simulink model "Linear_sys"  (R2024b)
settings: Solver=VariableStepAuto  StartTime=0.0  StopTime=300  RelTol=1e-3
settings Model: Creator=shalh  LastModifiedBy=shalh

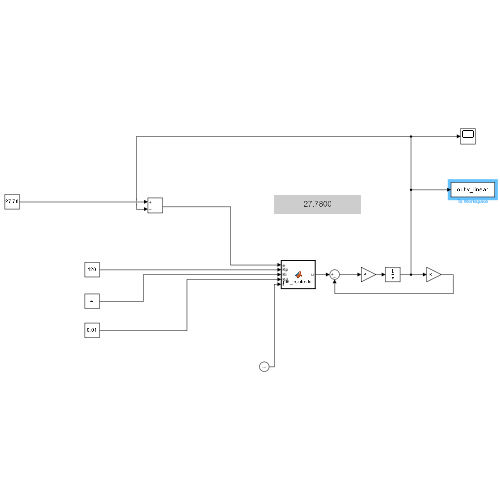
[thumbnail: Simulink's stored preview of the top-level diagram]
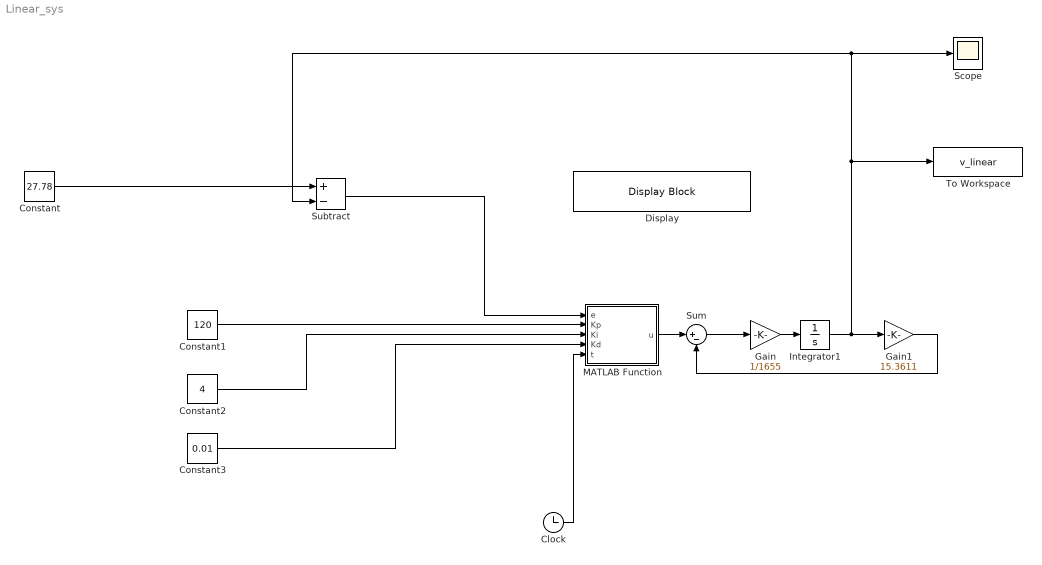
== system Linear_sys ==
  Clock : Clock
      settings: Decimation=40
  Constant : Constant  Value=27.78
  Constant1 : Constant  Value=120
  Constant2 : Constant  Value=4
  Constant3 : Constant  Value=0.01
  Display : DisplayBlock  LabelPosition=Hide  Transparency=1
  Gain : Gain  Gain=1/1655
  Gain1 : Gain  Gain=15.3611
  Integrator1 : Integrator
  MATLAB Function : MATLAB Function  TreatAsAtomicUnit=on
  Scope : Scope
  Subtract : Sum  Inputs=+-
  Sum : Sum  Inputs=|+-
  To Workspace : ToWorkspace  VariableName=v_linear  SampleTime=-1
  wires:
  Gain1/1 -> Sum/2
  Sum/1 -> Gain/1
  Constant3/1 -> MATLAB Function/4(Kd)
  Clock/1 -> MATLAB Function/5(t)
  Gain/1 -> Integrator1/1
  Subtract/1 -> MATLAB Function/1(e)
  Constant2/1 -> MATLAB Function/3(Ki)
  Constant1/1 -> MATLAB Function/2(Kp)
  MATLAB Function/1(u) -> Sum/1
  Constant/1 -> Subtract/1
  Integrator1/1 -> Scope/1, Subtract/2, To Workspace/1, Gain1/1

== matlab function Linear_sys/MATLAB Function ==
  settings: updateMethod=DISCRETE
  data: e input double; Kp input; Ki input; Kd input; u output double; t input
function u = pid_controller(e,Kp,Ki, Kd, t)
  
    persistent e_integral e_prev t_prev
    if isempty(e_integral)
        e_integral = 0;
        e_prev = 0;
        t_prev = 0;
    end
    
    
    if t_prev == 0
        dt = 0.01; 
    else
        dt = t - t_prev;
    end
    
    e_integral = e_integral + e * dt;
    
    if dt > 0
        e_derivative = (e - e_prev) / dt;
    else
        e_derivative = 0;
    end
    
    u = Kp * e + Ki * e_integral + Kd * e_derivative;
    
    e_prev = e;
    disp(e);
    t_prev = t;
end
